simulink model "QArmTestPWM"  (R2019a)
settings: Solver=ode4  StartTime=0.0  StopTime=inf  FixedStep=1/500  RelTol=1e-3  EnableMultiTasking=on
InitFcn:
  | home = [0.45; 0; 0.49];
  | pick = [0.66; 0; 0.3];
  | place = [-0.425; 0.5; 0.35];
  | midway_pick =  [ pick(1,1);  pick(2,1); home(3,1)];
  | midway_place = [0.5*place(1,1) + 0.5*home(1,1); 0.5*place(2,1) + 0.5*home(2,1); home(3,1)];
  | 
  | waypoints = ...
  | [pick,...
  | pick,...
  | place,...
  | place,...
  | home]' ;
undefined symbols (not defined in the file): HIL
libraries: quarc_library x4
settings Model: ExtModeTrigDuration=10000  Creator=fvranes  LastModifiedBy=mbohra
settings SolverCC: PositivePriorityOrder=on
settings DataIOCC: ReturnWorkspaceOutputs=off
settings OptimizationCC: LifeSpan=inf
settings DebuggingCC: ArithmeticOperatorsInVariantConditions=warning
settings SFSimCC: SimUseLocalCustomCode=off
settings RTWCC: SystemTargetFile=quarc_win64.tlc  TemplateMakefile=quarc_default_tmf  Description=QUARC Win64 Target  RTWUseLocalCustomCode=off
settings CodeAppCC: StateflowObjectComments=on
settings STFCustomTargetCC: TargetPreCompLibLocation=C:\PROGRA~3\QUARC\lib\2019a\win64\debug  TargetLangStandard=C99 (ISO)  ConcurrentExecutionCompliant=on  SystemTargetFile=quarc_win64.tlc
settings GRTTargetCC: TargetPreCompLibLocation=C:\PROGRA~3\QUARC\lib\2019a\win64\debug  ParMdlRefBuildCompliant=off  CompOptLevelCompliant=off  CombineOutputUpdateFcns=off  MatFileLogging=off  CPPClassGenCompliant=off  GRTInterface=on  UseToolchainInfoCompliant=off  ExtMode=on  ExtModeMexFile=quarc_comm
settings ConfigComp: CovMetricSettings=dswe

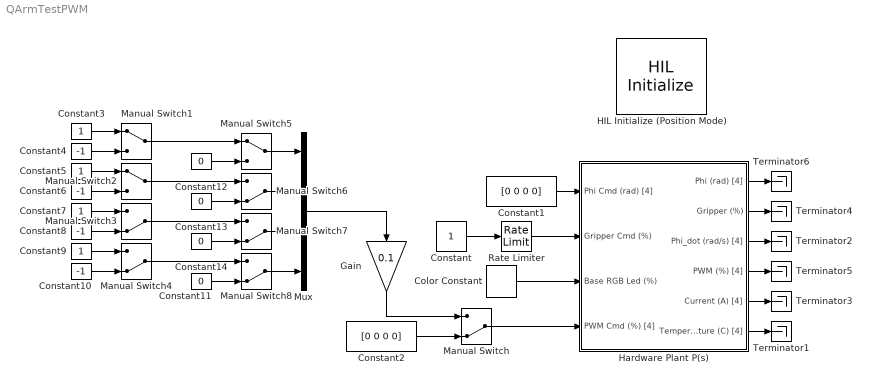
== system QArmTestPWM ==
  Color Constant : quarc_library/Sources/Signals/Color Constant  color=[0.71765 0.27451 1]
      settings: SourceProductName=QUARC Targets
  Constant : Constant
  Constant1 : Constant  Value=[0 0 0 0]
  Constant{4,6,8,10} (4 alike) : Constant  Value=-1  VectorParams1D=off
  Constant{11..14} (4 alike) : Constant  Value=0  VectorParams1D=off
  Constant2 : Constant  Value=[0 0 0 0]
  Constant{3,5,7,9} (4 alike) : Constant  VectorParams1D=off
  Gain : Gain  Gain=0.1
  HIL Initialize (Position Mode) : quarc_library/Data Acquisition/Generic/Configuration/HIL Initialize  object_name=HIL-1  board_type=qarm_usb  board_number=0@tcpip://localhost:18900?nagle='off'  board_options=qbus_clk_divisor=6;sync_timer_period=160000;sync_timer_threshold=26200;j0_mode=1;j1_mode=1;j2_mode=1;j3_mode=1;gripper_mode=0;j0_profile_config=0;j0_profile_velocity=0;j0_profile_acceleration=0;j1_profile_config=0;j1_profile_velocity=0;j1_profile_acceleration=0;j2_profile_config=0;j2_profile_velocity=0;j2_profile_acceleration=0;j3_profile_config=0;j3_profile_velocity=0;j3_profile_acceleration=0;gripper_profile_config=0;gripper_profile_velocity=0;gripper_profile_acceleration=0;  exclusive=off  active=on  hardware_clocks=[0]  clock_modes=[]  initial_clock_frequencies=[]  set_clock_params_at_start=off  set_clock_params_at_switch_in=off  set_clock_frequencies_at_start=off  set_clock_frequencies_at_switch_in=off  analog_input_channels=[5:9]  analog_input_configurations=[]  analog_input_maximums=[]  analog_input_minimums=[]  set_analog_input_params_at_start=off  set_analog_input_params_at_switch_in=off  analog_output_channels=[]  analog_output_maximums=inf  analog_output_minimums=-inf  initial_analog_outputs=[0]  final_analog_outputs=[0]  watchdog_analog_outputs=[]  set_analog_output_params_at_start=off  set_analog_output_params_at_switch_in=off  set_analog_outputs_at_start=off  set_analog_outputs_at_switch_in=off  set_analog_outputs_at_terminate=off  set_analog_outputs_at_switch_out=off  set_analog_outputs_on_watchdog=off  digital_input_channels=[]  digital_output_channels=[]  digital_output_configuration=[]  initial_digital_outputs=[0]  final_digital_outputs=[0]  watchdog_digital_outputs=[0]  set_digital_output_params_at_start=off  set_digital_output_params_at_switch_in=off  set_digital_outputs_at_start=off  set_digital_outputs_at_switch_in=off  set_digital_outputs_at_terminate=off  set_digital_outputs_at_switch_out=off  set_digital_outputs_on_watchdog=off  encoder_channels=[]  quadrature=[]  encoder_filter_frequency=[]  initial_encoder_counts=[]  set_encoder_params_at_start=off  set_encoder_params_at_switch_in=off  set_encoder_counts_at_start=off  set_encoder_counts_at_switch_in=off  pwm_channels=[]  pwm_modes=[]  pwm_frequency=[]  pwm_configuration=[]  pwm_alignment=[]  pwm_polarity=[]  pwm_leading_deadband=[]  pwm_trailing_deadband=[]  initial_pwm_outputs=[]  final_pwm_outputs=[]  watchdog_pwm_outputs=[]  set_pwm_params_at_start=off  set_pwm_params_at_switch_in=off  set_pwm_outputs_at_start=off  set_pwm_outputs_at_switch_in=off  set_pwm_outputs_at_terminate=off  set_pwm_outputs_at_switch_out=off  set_pwm_outputs_on_watchdog=off  other_output_channels=[1000:1004 11000:11003 11005:11007]  initial_other_outputs=[zeros(1,9), ones(1,3)]  final_other_outputs=[zeros(1,9), ones(1,3)]  watchdog_other_outputs=zeros(1,12)  set_other_outputs_at_start=off  set_other_outputs_at_switch_in=off  set_other_outputs_at_terminate=on  set_other_outputs_at_switch_out=off  set_other_outputs_on_watchdog=off
  Hardware Plant P(s) : Subsystem
  Manual Switch{,3..4,6..8} (6 alike) : ManualSwitch  CurrentSetting=0
  Manual Switch1 : ManualSwitch
  Manual Switch2 : ManualSwitch
  Manual Switch5 : ManualSwitch
  Mux : Mux
  Rate Limiter : RateLimiter  SampleTimeMode=inherited
  Terminator{1..6} (6 alike) : Terminator
  wires:
  Hardware Plant P(s)/4(PWM (%) [4]) -> Terminator5/1
  Hardware Plant P(s)/3(Phi_dot (rad/s) [4]) -> Terminator2/1
  Hardware Plant P(s)/6(Temperature (C) [4]) -> Terminator1/1
  Rate Limiter/1 -> Hardware Plant P(s)/2(Gripper Cmd (%))
  Hardware Plant P(s)/5(Current (A) [4]) -> Terminator3/1
  Color Constant/1 -> Hardware Plant P(s)/3(Base RGB Led (%))
  Manual Switch/1 -> Hardware Plant P(s)/4(PWM Cmd (%) [4])
  Constant/1 -> Rate Limiter/1
  Hardware Plant P(s)/2(Gripper (%)) -> Terminator4/1
  Constant1/1 -> Hardware Plant P(s)/1(Phi Cmd (rad) [4])
  Constant2/1 -> Manual Switch/2
  Constant4/1 -> Manual Switch1/2
  Constant3/1 -> Manual Switch1/1
  Constant5/1 -> Manual Switch2/1
  Constant6/1 -> Manual Switch2/2
  Constant10/1 -> Manual Switch4/2
  Constant9/1 -> Manual Switch4/1
  Constant7/1 -> Manual Switch3/1
  Constant8/1 -> Manual Switch3/2
  Mux/1 -> Gain/1
  Gain/1 -> Manual Switch/1
  Constant12/1 -> Manual Switch5/2
  Constant13/1 -> Manual Switch6/2
  Constant14/1 -> Manual Switch7/2
  Constant11/1 -> Manual Switch8/2
  Manual Switch4/1 -> Manual Switch8/1
  Manual Switch3/1 -> Manual Switch7/1
  Manual Switch2/1 -> Manual Switch6/1
  Manual Switch1/1 -> Manual Switch5/1
  Manual Switch5/1 -> Mux/1
  Manual Switch6/1 -> Mux/2
  Manual Switch7/1 -> Mux/3
  Manual Switch8/1 -> Mux/4
  Hardware Plant P(s)/1(Phi (rad) [4]) -> Terminator6/1

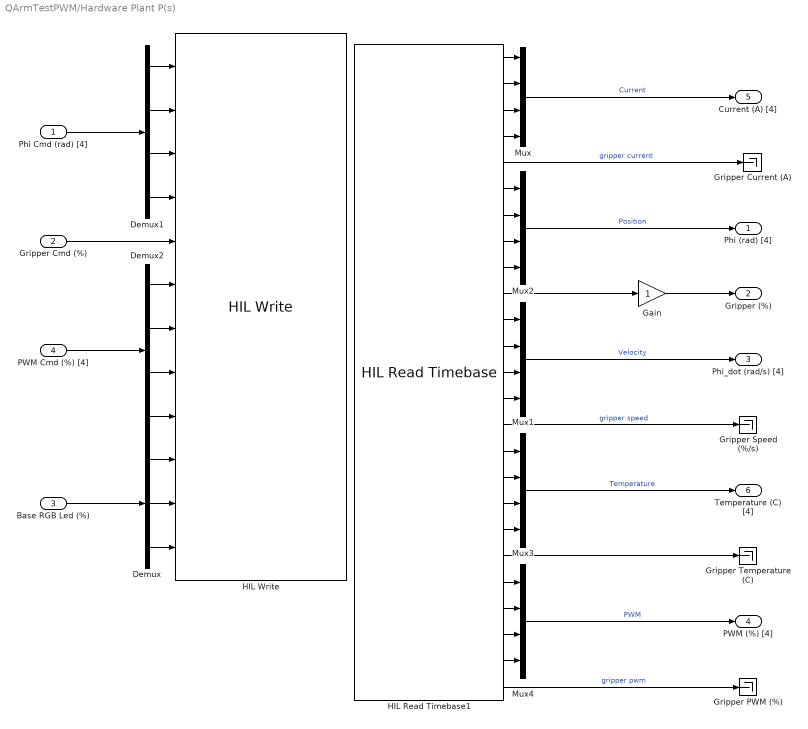
== system QArmTestPWM/Hardware Plant P(s) ==
  Phi Cmd (rad) [4] : Inport
  Gripper Cmd (%) : Inport  Port=2
  Base RGB Led (%) : Inport  Port=3
  PWM Cmd (%) [4] : Inport  Port=4
  Demux : Demux  Outputs=3
  Demux1 : Demux
  Demux2 : Demux
  Gain : Gain
  Gripper Current (A) : Terminator
  Gripper PWM (%) : Terminator
  Gripper Speed (%/s) : Terminator
  Gripper Temperature (C) : Terminator
  HIL Read Timebase1 : quarc_library/Data Acquisition/Generic/Timebases/HIL Read Timebase  object_name=HIL-1  clock=0  analog_channels=[5:9]  encoder_channels=[]  digital_channels=[]  other_channels=[1000:1004 3000:3004 10000:10004 11000:11004]  active=on  vector_output=off  data_type_mode=Inherit via back propagation  encoder_data_type=double  digital_data_type=boolean  overflow_mode=Wait on overflow (for simulated cards only)  samples_in_buffer=1
  HIL Write : quarc_library/Data Acquisition/Generic/Immediate I//O/HIL Write  object_name=HIL-1  analog_channels=[]  pwm_channels=[]  digital_channels=[]  other_channels=[1000:1004 11000:11003 11005:11007]  sample_time=-1  active=on  vector_input=off
  Mux{,1..4} (5 alike) : Mux
  Phi (rad) [4] : Outport
  Gripper (%) : Outport  Port=2
  Phi_dot (rad/s) [4] : Outport  Port=3
  PWM (%) [4] : Outport  Port=4
  Current (A) [4] : Outport  Port=5
  Temperature (C) [4] : Outport  Port=6
  wires:
  HIL Read Timebase1/14 -> Mux1/4
  HIL Read Timebase1/9 -> Mux2/4
  HIL Read Timebase1/6 -> Mux2/1
  HIL Read Timebase1/18 -> Mux3/3
  HIL Read Timebase1/8 -> Mux2/3
  HIL Read Timebase1/12 -> Mux1/2
  HIL Read Timebase1/4 -> Mux/4
  HIL Read Timebase1/7 -> Mux2/2
  HIL Read Timebase1/5 -> Gripper Current (A)/1  "gripper current"
  HIL Read Timebase1/15 -> Gripper Speed (%/s)/1  "gripper speed"
  Demux/3 -> HIL Write/12
  HIL Read Timebase1/3 -> Mux/3
  HIL Read Timebase1/17 -> Mux3/2
  HIL Read Timebase1/16 -> Mux3/1
  HIL Read Timebase1/11 -> Mux1/1
  Demux/1 -> HIL Write/10
  HIL Read Timebase1/19 -> Mux3/4
  Demux/2 -> HIL Write/11
  HIL Read Timebase1/13 -> Mux1/3
  HIL Read Timebase1/2 -> Mux/2
  HIL Read Timebase1/1 -> Mux/1
  HIL Read Timebase1/20 -> Gripper Temperature (C)/1
  Mux/1 -> Current (A) [4]/1  "Current"
  Mux1/1 -> Phi_dot (rad/s) [4]/1  "Velocity"
  Mux3/1 -> Temperature (C) [4]/1  "Temperature"
  Base RGB Led (%)/1 -> Demux/1
  Demux1/1 -> HIL Write/1
  Demux1/2 -> HIL Write/2
  Demux1/3 -> HIL Write/3
  Demux1/4 -> HIL Write/4
  Phi Cmd (rad) [4]/1 -> Demux1/1
  PWM Cmd (%) [4]/1 -> Demux2/1
  Demux2/1 -> HIL Write/6
  Demux2/2 -> HIL Write/7
  Demux2/3 -> HIL Write/8
  Demux2/4 -> HIL Write/9
  Mux2/1 -> Phi (rad) [4]/1  "Position"
  HIL Read Timebase1/21 -> Mux4/1
  HIL Read Timebase1/22 -> Mux4/2
  HIL Read Timebase1/23 -> Mux4/3
  HIL Read Timebase1/24 -> Mux4/4
  HIL Read Timebase1/25 -> Gripper PWM (%)/1  "gripper pwm"
  Mux4/1 -> PWM (%) [4]/1  "PWM"
  HIL Read Timebase1/10 -> Gain/1
  Gain/1 -> Gripper (%)/1
  Gripper Cmd (%)/1 -> HIL Write/5
